simulink model "persistent_test_m"  (R2020b)
settings: Solver=VariableStepAuto  StartTime=0.0  StopTime=stop_time  FixedStep=Ts  MaxStep=0.001  RelTol=1e-3
values from neighbouring files (symbols this model uses):
  T_filtr = 0.1    [persistent_test.m]
  Ts = 0.001    [persistent_test.m]
libraries: simulink x1
settings Model: Creator=Adam  LastModifiedBy=Adam
settings DebuggingCC: AlgebraicLoopMsg=none

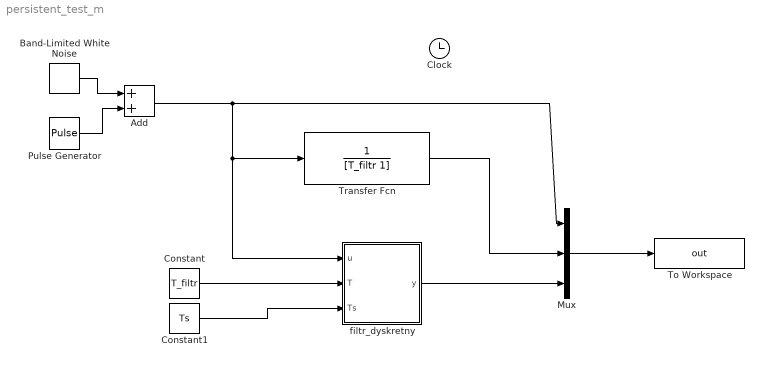
== system persistent_test_m ==
  Add : Sum
  Band-Limited White Noise : simulink/Sources/Band-Limited White Noise  Cov=[0.000001]  Ts=Ts  seed=[23341]
  Clock : Clock
  Constant : Constant  Value=T_filtr
  Constant1 : Constant  Value=Ts
  Mux : Mux  Inputs=3
  Pulse Generator : DiscretePulseGenerator  PulseType=Time based  Period=10  PulseWidth=50
  To Workspace : ToWorkspace  VariableName=out  SaveFormat=Structure  SampleTime=-1
      settings: Save2DSignal=2-D array (concatenate along first dimension)
  Transfer Fcn : TransferFcn  Denominator=[T_filtr 1]
  filtr_dyskretny : MATLAB Function  TreatAsAtomicUnit=on  SystemSampleTime=Ts
  wires:
  Band-Limited White Noise/1 -> Add/1
  Pulse Generator/1 -> Add/2
  Add/1 -> filtr_dyskretny/1(u), Transfer Fcn/1, Mux/1
  Transfer Fcn/1 -> Mux/2
  filtr_dyskretny/1(y) -> Mux/3
  Constant/1 -> filtr_dyskretny/2(T)
  Constant1/1 -> filtr_dyskretny/3(Ts)
  Mux/1 -> To Workspace/1

== matlab function persistent_test_m/filtr_dyskretny ==
  data: u input; y output; T input; Ts input
function y = filter(u, T, Ts)
%% stale parametry
limit = 10;

%%
persistent x x_pop u_pop

if isempty(x)
    x_pop = 0;
    u_pop = 0;
end

%% kod filtru
x = -x_pop * (Ts - 2*T) / (2*T + Ts) + ...
    u*Ts/(2*T + Ts) + u_pop * Ts / (2*T + Ts);

%% saturacja i przesuwanie próbek
if abs(x) >= limit
    x = sign(x) * limit;
else
    x = x;
end

x_pop = x;
u_pop = u;

y = x;

end
